simulink model "task1_2"  (R2019b)
settings: Solver=VariableStepAuto  StartTime=0.0  StopTime=2  RelTol=1e-3
settings Model: EnablePacing=on  PacingRate=0.140000  Creator=HUAWEI  LastModifiedBy=HUAWEI

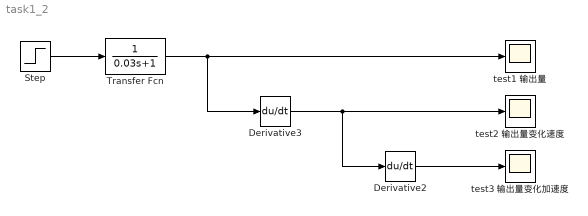
== system task1_2 ==
  Derivative2 : Derivative
  Derivative3 : Derivative
  Step : Step  Time=0.1  SampleTime=0
  Transfer Fcn : TransferFcn  Denominator=[0.03 1]
  test1 输出量 : Scope
  test2 输出量变化速度 : Scope
  test3 输出量变化加速度 : Scope
  wires:
  Transfer Fcn/1 -> test1 输出量/1, Derivative3/1
  Derivative3/1 -> Derivative2/1, test2 输出量变化速度/1
  Derivative2/1 -> test3 输出量变化加速度/1
  Step/1 -> Transfer Fcn/1
